simulink model "three_phase_WPT"  (R2020b)
settings: Solver=FixedStepDiscrete  StartTime=0.0  StopTime=Tfinal  FixedStep=SampleTime  RelTol=1e-3
InitFcn:
  | param
values from neighbouring files (symbols this model uses):
  C_DCA = 1e-6    (= 1e-06)    [param.m]
  C_DCB = 1e-6    (= 1e-06)    [param.m]
  C_DCC = 1e-6    (= 1e-06)    [param.m]
  Cp = 1.7349e-08    [param.m]
  Cs = 5.9683e-08    [param.m]
  ESRA = 1e-7    (= 1e-07)    [param.m]
  ESRB = 1e-7    (= 1e-07)    [param.m]
  ESRC = 1e-7    (= 1e-07)    [param.m]
  f_motor = 300    [param.m]
  LA_mid_parasitic = 1e-8    (= 1e-08)    [param.m]
  LA_parasitic = 1e-8    (= 1e-08)    [param.m]
  LAB_parasitic = 1e-8    (= 1e-08)    [param.m]
  LB_mid_parasitic = 1e-8    (= 1e-08)    [param.m]
  LB_parasitic = 1e-8    (= 1e-08)    [param.m]
  LBC_parasitic = 1e-8    (= 1e-08)    [param.m]
  LC_mid_parasitic = 1e-8    (= 1e-08)    [param.m]
  LC_parasitic = 1e-8    (= 1e-08)    [param.m]
  Lp = 2.2813e-04    (= 0.00022813)    [param.m]
  Ls = 6.6315e-05    [param.m]
  LSource = 1e-6    (= 1e-06)    [param.m]
  M = 1.8450e-05    (= 1.845e-05)    [param.m]
  ma = 0:0.01:1    [analitik_calculation.m]    (also in analytical_v2.m; param.m = 0.9)
  RA_mid_parasitic = 1e-3    (= 0.001)    [param.m]
  RA_parasitic = 1e-3    (= 0.001)    [param.m]
  RAB_parasitic = 1e-3    (= 0.001)    [param.m]
  RB_mid_parasitic = 1e-3    (= 0.001)    [param.m]
  RBC_parasitic = 1e-3    (= 0.001)    [param.m]
  RC_mid_parasitic = 1e-3    (= 0.001)    [param.m]
  RL = 8.33*1.2337    (= 10.276721)    [param.m]
  RSource = 0.1    [param.m]
  SampleTime = 1e-8    (= 1e-08)    [param.m]
  Tfinal = 0.05    [param.m]
  VDC = 200    [param.m]
undefined symbols (not defined in the file or in its folder): C_DC, ESLA, ESLB
libraries: powerlib x100, eeStairGenerator x2, eeGeneralControl x1
settings Model: Creator=enes_  LastModifiedBy=enes_
settings DataIOCC: ReturnWorkspaceOutputs=off
settings DebuggingCC: ArithmeticOperatorsInVariantConditions=warning
settings SFSimCC: SimUseLocalCustomCode=off  CustomCodeUndefinedFunction=UseInterfaceOnly
settings RTWCC: RTWUseLocalCustomCode=off

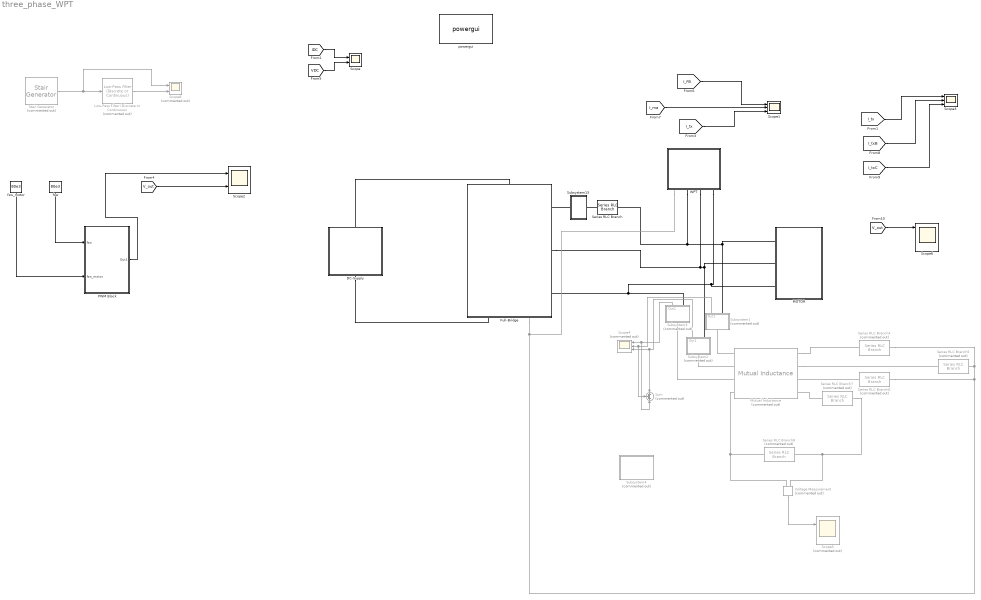
== system three_phase_WPT ==
  DC-Supply : Subsystem
  Full-Bridge : Subsystem
      settings: PortSchema="{\"entries\":[{\"content\":{\"sides\":[{\"content\":{\"connectorIds\":[]},\"type\":\"ConnectorPlacement.EquallySpacedRectSide\",\"uuid\":\"92c2640b-bb56-47f8-9c41-2323b38839f8\"},{\"content\":{\"connectorIds\":[\"RConn1\",\"RConn2\",\"RConn3\"],\"side\":\"RIGHT\"},\"type\":\"ConnectorPlacement.EquallySpacedRectSide\",\"uuid\":\"0b5c90a1-e2e1-4478-84c9-834496a6568e\"},{\"content\":{\"connectorIds\":[\"LConn1\"],\"side\":\"TOP\"},\"type\":\"ConnectorPlacement.EquallySpacedRectSide\",\"uuid\":\"1c803fb0-9096-4a7d-b495-aabd35d72306\"},{\"content\":{\"connectorIds\":[\"RConn4\",\"RConn5\"],\"side\":\"BOTTOM\"},\"type\":\"ConnectorPlacement.EquallySpacedRectSide\",\"uuid\":\"5a2d766c-8c3f-4943-ab0f-0e1988e2f8d8\"},{\"content\":{\"connectorIds\":[],\"side\":\"HIDDEN\"},\"type\":\"ConnectorPlacement.EquallySpacedRectSide\",\"uuid\":\"8868c32c-a67f-4887-a91d-dc24242eaee2\"}]},\"type\":\"ConnectorPlacement.EquallySpacedConnector\",\"uuid\":\"a3546067-6216-40b0-bae0-9d71271c5112\"}],\"packageUris\":[\"http://schema.mathworks.com/mf0/Connector/R2020b\"],\"version\":\"1.0\"}"
  Low-Pass Filter (Discrete or Continuous) : eeGeneralControl/Low-Pass Filter (Discrete or Continuous)  Commented=on  K=1  T=2e-3  B=inf  A=-inf  init_option=Inherited from block input  x0=0  Ts=-1
  MOTOR : Subsystem
      settings: PortSchema="{\"entries\":[{\"content\":{\"sides\":[{\"content\":{\"connectorIds\":[]},\"type\":\"ConnectorPlacement.EquallySpacedRectSide\",\"uuid\":\"27af0988-5d70-46f2-9f63-66e4679735d7\"},{\"content\":{\"connectorIds\":[],\"side\":\"RIGHT\"},\"type\":\"ConnectorPlacement.EquallySpacedRectSide\",\"uuid\":\"9d673fb6-38db-4110-ad66-771dcf318fba\"},{\"content\":{\"connectorIds\":[\"LConn1\",\"LConn2\",\"LConn3\"],\"side\":\"TOP\"},\"type\":\"ConnectorPlacement.EquallySpacedRectSide\",\"uuid\":\"44eb7bd4-c702-4f50-84c2-cb9d75020b5b\"},{\"content\":{\"connectorIds\":[],\"side\":\"HIDDEN\"},\"type\":\"ConnectorPlacement.EquallySpacedRectSide\",\"uuid\":\"ba714e9b-5efc-4dbb-add8-803f06cf9de0\"}]},\"type\":\"ConnectorPlacement.EquallySpacedConnector\",\"uuid\":\"a2219d53-abb4-437b-a840-c37860cec52f\"}],\"packageUris\":[\"http://schema.mathworks.com/mf0/Connector/R2020b\"],\"version\":\"1.0\"}"
  Mutual Inductance : powerlib/Elements/Mutual Inductance  Commented=on  LConnTagsString=a|b|c|L4  RConnTagsString=A|B|C|R4  TypeOfMutual=Generalized mutual inductance  NumberOfWindings=4  SelfImpedance1=[1.1 1.1e-03]  SelfImpedance2=[ 1.1 1.1e-03]  ThreeWindings=on  SelfImpedance3=[ 1.1 1.1e-03]  MutualImpedance=[1.0 1.0e-03]  InductanceMatrix="[1 0  0 0.2 ;  0 1  0 0.2 ;0 0  1 0.2 ;0.2 0.2  0.2 1  ] * 1e-3"  ResistanceMatrix="[ 1  0 0 0 ;  0 1 0 0 ; 0 0 1 0  ;0 0 0 1 ]"  Measurements=Winding currents
      settings: AttributesFormatString=\n  SourceProductBaseCode=PS
  PWM Block : Subsystem
  Scope : Scope  NumInputPorts=2
  Scope1 : Scope  NumInputPorts=3
  Scope2 : Scope  NumInputPorts=2
  Scope3 : Scope  NumInputPorts=3
  Scope4 : Scope  Commented=on  NumInputPorts=3
  Scope5 : Scope  Commented=on  NumInputPorts=2
  Scope6 : Scope  NumInputPorts=3
  Scope8 : Scope  Commented=on  NumInputPorts=2
  Series RLC Branch : powerlib/Elements/Series RLC Branch  LConnTagsString=__new0  RConnTagsString=__new0  BranchType=RL  Resistance=1e-2  Inductance=1e-6  SetiL0=off  InitialCurrent=0  Capacitance=1e-6  Setx0=off  InitialVoltage=0  Measurements=None
  Series RLC Branch4 : powerlib/Elements/Series RLC Branch  Commented=on  LConnTagsString=__new0  RConnTagsString=__new0  BranchType=C  Resistance=1  Inductance=1e-3  SetiL0=off  InitialCurrent=0  Capacitance=3.9579e-09  Setx0=off  InitialVoltage=0  Measurements=None
  Series RLC Branch5 : powerlib/Elements/Series RLC Branch  Commented=on  LConnTagsString=__new0  RConnTagsString=__new0  BranchType=C  Resistance=1  Inductance=1e-3  SetiL0=off  InitialCurrent=0  Capacitance=3.9579e-09  Setx0=off  InitialVoltage=0  Measurements=None
  Series RLC Branch6 : powerlib/Elements/Series RLC Branch  Commented=on  LConnTagsString=__new0  RConnTagsString=__new0  BranchType=C  Resistance=1  Inductance=1e-3  SetiL0=off  InitialCurrent=0  Capacitance=3.9579e-09  Setx0=off  InitialVoltage=0  Measurements=None
  Series RLC Branch7 : powerlib/Elements/Series RLC Branch  Commented=on  LConnTagsString=__new0  RConnTagsString=__new0  BranchType=C  Resistance=1  Inductance=1e-3  SetiL0=off  InitialCurrent=0  Capacitance=Cs  Setx0=off  InitialVoltage=0  Measurements=None
  Series RLC Branch8 : powerlib/Elements/Series RLC Branch  Commented=on  LConnTagsString=__new0  RConnTagsString=__new0  BranchType=R  Resistance=10  Inductance=1e-3  SetiL0=off  InitialCurrent=0  Capacitance=Cs  Setx0=off  InitialVoltage=0  Measurements=None
  Stair Generator : eeStairGenerator/Stair Generator  Commented=on  LabelModeActiveChoice=Discrete  TimeInput=Tfinal*[0 1/4 2/4 3/4 ]  AmplitudeInput=[0.50 0.8 0.6 0.5 ]  SampleTime=-1  RepeatPattern=off  OutDataTypeStr=double
      settings: SourceProductBaseCode=PS
  Subsystem1 : Subsystem  Commented=on
  Subsystem13 : Subsystem
  Subsystem2 : Subsystem  Commented=on
  Subsystem3 : Subsystem  Commented=on
  Subsystem4 : Subsystem  Commented=on
  Sum : Sum  Commented=on  Inputs=+++
  Voltage Measurement : powerlib/Measurements/Voltage Measurement  Commented=on  PhasorSimulation=off  OutputType=Complex  PSBequivalent=0
  WPT : Subsystem
  fsw : Constant  Value=80e3
  fsw_motor : Constant  Value=80e3
  powergui : powerlib/powergui  Priority=1  SimulationMode=Discrete  SampleTime=SampleTime  frequency=60  Iterations=50  frequencyindice=0  Pbase=100e6  ErrMax=1e-4  UnitsV=kV  UnitsW=MW  buscounter=0  FunctionMessages=off  echomessages=off  EnableUseOfTLC=off  CurrentSourceSwitches=off  DisableSnubberDevices=off  DisableRonSwitches=off  DisableVfSwitches=off  DisplayEquations=off  AutomaticDiscreteSolvers=off  SolverType=Tustin/Backward Euler (TBE)  Interpol=off  ExternalGateDelay=off  methode=off  Ts=100  x0status=blocks  SPID=on  SwTol=0  HookPort=off  NonlinearTolerance=1e-4  nMaxIteration=100  ContinueOnMaxIteration=off  RestoreLinks=warning  ResistiveCurrentMeasurement=off  Frange=[1e3:1e3:240e3]  Ylog=off  Xlog=on  ShowGrid=off  save=off  variable=ZData  structure=ScopeData2  ZoomFFT=off  StartTime=0.02  cycles=400  DisplayStyle=2  fundamental=80e3  FreqAxis=off  MaxFrequency=240e3  frequencyindicesteady=1  RmsSteady=1  display=off
  wires:
  Low-Pass Filter (Discrete or Continuous)/1 -> Scope8/2
  [IDC] -> Scope/1
  [VDC] -> Scope/2
  [I_FB] -> Scope1/1
  [I_ma] -> Scope1/2
  [I_tx] -> Scope1/3
  Stair Generator/1 -> Scope8/1, Low-Pass Filter (Discrete or Continuous)/1
  fsw_motor/1 -> PWM Block/2(fsw_motor)
  [V_out] -> Scope2/2
  PWM Block/1(Out1) -> Scope2/1
  fsw/1 -> PWM Block/1(fsw)
  [I_tx] -> Scope3/1
  [I_txB] -> Scope3/2
  [I_txC] -> Scope3/3
  Subsystem3/1(Out1) -> Sum/3, Scope4/1
  Subsystem1/1(Out1) -> Sum/2, Scope4/2
  Subsystem2/1(Out1) -> Sum/1, Scope4/3
  Voltage Measurement/1 -> Scope5/1
  [V_out] -> Scope6/1
  connections:
  DC-Supply/LConn1 -- Full-Bridge/LConn1
  DC-Supply/RConn1 -- Full-Bridge/RConn4
  Series RLC Branch/LConn1 -- Subsystem13/LConn1
  Subsystem13/RConn1 -- Full-Bridge/RConn1
  Full-Bridge/RConn2 -- WPT/LConn2 -- Subsystem2/RConn1 -- MOTOR/LConn2
  Mutual Inductance/RConn2 -- Series RLC Branch5/RConn1
  Series RLC Branch6/RConn1 -- Mutual Inductance/RConn3
  Series RLC Branch7/RConn1 -- Mutual Inductance/RConn4
  Voltage Measurement/LConn1 -- Series RLC Branch7/LConn1 -- Series RLC Branch8/LConn1
  MOTOR/LConn1 -- Series RLC Branch/RConn1 -- WPT/LConn3 -- Subsystem1/RConn1
  Subsystem2/LConn1 -- Mutual Inductance/LConn2
  MOTOR/LConn3 -- WPT/LConn1 -- Full-Bridge/RConn3 -- Subsystem3/RConn1
  Subsystem3/LConn1 -- Mutual Inductance/LConn3
  Mutual Inductance/LConn1 -- Subsystem1/LConn1
  Mutual Inductance/RConn1 -- Series RLC Branch4/RConn1
  Series RLC Branch6/LConn1 -- WPT/LConn4 -- Full-Bridge/RConn5 -- Series RLC Branch4/LConn1 -- Series RLC Branch5/LConn1
  Voltage Measurement/LConn2 -- Mutual Inductance/LConn4 -- Series RLC Branch8/RConn1

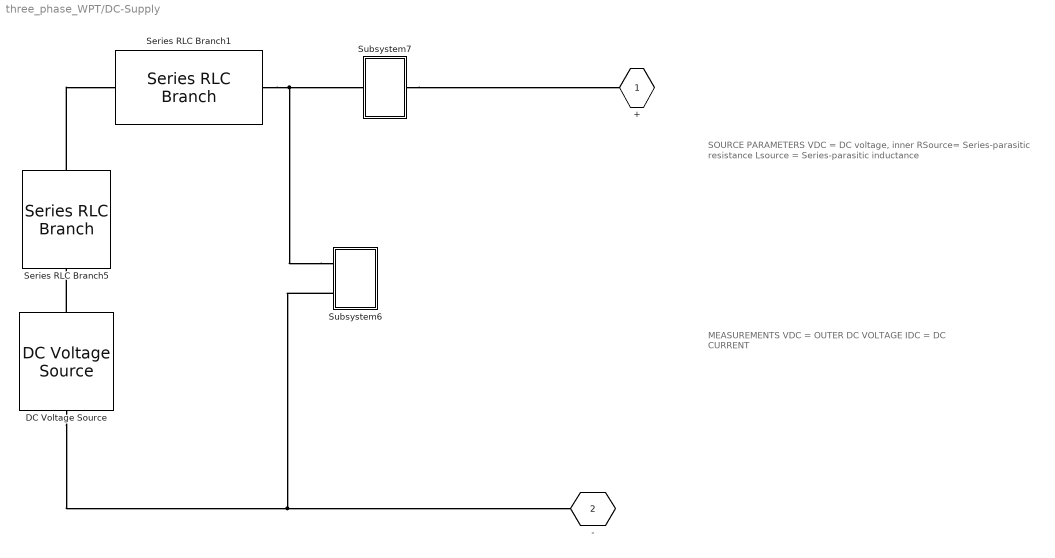
== system three_phase_WPT/DC-Supply ==
  note: SOURCE PARAMETERS
      | VDC = DC voltage, inner
      | RSource= Series-parasitic resistance
      | Lsource = Series-parasitic inductance
  note: MEASUREMENTS
      | VDC = OUTER DC VOLTAGE
      | IDC = DC CURRENT
  DC Voltage Source : powerlib/Electrical Sources/DC Voltage Source  Amplitude=VDC  Measurements=None
  Series RLC Branch1 : powerlib/Elements/Series RLC Branch  LConnTagsString=__new0  RConnTagsString=__new0  BranchType=L  Resistance=LSource  Inductance=LSource  SetiL0=off  InitialCurrent=0  Capacitance=0.01  Setx0=off  InitialVoltage=0  Measurements=None
  Series RLC Branch5 : powerlib/Elements/Series RLC Branch  LConnTagsString=__new0  RConnTagsString=__new0  BranchType=R  Resistance=RSource  Inductance=ESLA  SetiL0=off  InitialCurrent=0  Capacitance=0.01  Setx0=off  InitialVoltage=0  Measurements=None
  Subsystem6 : Subsystem
  Subsystem7 : Subsystem
  + : PMIOPort  Side=Left
  - : PMIOPort  Port=2  Side=Right
  connections:
  Series RLC Branch5/LConn1 -- Series RLC Branch1/RConn1
  DC Voltage Source/LConn1 -- Subsystem6/LConn2 -- -/RConn1
  Subsystem6/LConn1 -- Subsystem7/RConn1 -- Series RLC Branch1/LConn1
  DC Voltage Source/RConn1 -- Series RLC Branch5/RConn1
  Subsystem7/LConn1 -- +/RConn1

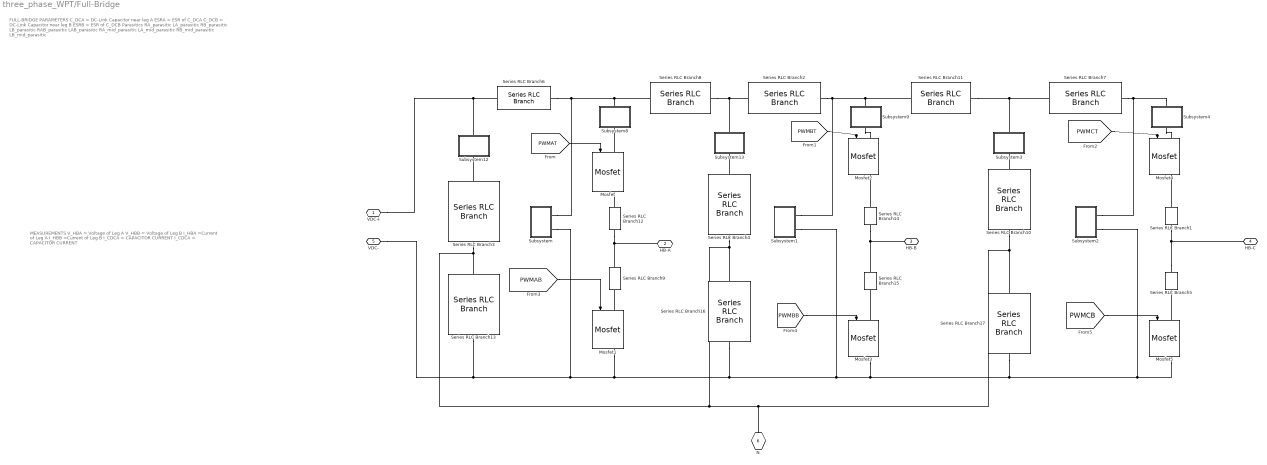
== system three_phase_WPT/Full-Bridge ==
  note: MEASUREMENTS
      | V_HBA = Voltage of Leg A
      | V_HBB = Voltage of Leg B
      | I_HBA =Current of Leg A
      | I_HBB =Current of Leg B
      | I_CDCA = CAPACITOR CURRENT
      | I_CDCA = CAPACITOR CURRENT
  note: FULL-BRIDGE PARAMETERS
      | C_DCA = DC-Link Capacitor near leg A
      | ESRA = ESR of C_DCA
      | C_DCB = DC-Link Capacitor near leg B
      | ESRB = ESR of C_DCB
      | Parasitics
      | RA_parasitic
      | LA_parasitic
      | RB_parasitic
      | LB_parasitic
      | RAB_parasitic
      | LAB_parasitic
      | RA_mid_parasitic
      | LA_mid_parasitic
      | RB_mid_parasitic
      | LB_mid_parasitic
  Mosfet{,1..5} (6 alike) : powerlib/Power Electronics/Mosfet  Ron=0.1  Lon=0  Rd=0.01  Vfd=0  IC=0  Rs=1e5  Cs=inf  Measurements=on
  Series RLC Branch1 : powerlib/Elements/Series RLC Branch  LConnTagsString=__new0  RConnTagsString=__new0  BranchType=RL  Resistance=RC_mid_parasitic  Inductance=LC_mid_parasitic  SetiL0=off  InitialCurrent=0  Capacitance=C_DC  Setx0=off  InitialVoltage=0  Measurements=None
  Series RLC Branch10 : powerlib/Elements/Series RLC Branch  LConnTagsString=__new0  RConnTagsString=__new0  BranchType=RC  Resistance=ESRC  Inductance=ESLB  SetiL0=off  InitialCurrent=0  Capacitance=C_DCC  Setx0=off  InitialVoltage=0  Measurements=None
  Series RLC Branch11 : powerlib/Elements/Series RLC Branch  LConnTagsString=__new0  RConnTagsString=__new0  BranchType=RL  Resistance=RBC_parasitic  Inductance=LBC_parasitic  SetiL0=off  InitialCurrent=0  Capacitance=0.01  Setx0=off  InitialVoltage=0  Measurements=None
  Series RLC Branch12 : powerlib/Elements/Series RLC Branch  LConnTagsString=__new0  RConnTagsString=__new0  BranchType=RL  Resistance=RA_mid_parasitic  Inductance=LA_mid_parasitic  SetiL0=off  InitialCurrent=0  Capacitance=C_DC  Setx0=off  InitialVoltage=0  Measurements=None
  Series RLC Branch13 : powerlib/Elements/Series RLC Branch  LConnTagsString=__new0  RConnTagsString=__new0  BranchType=RC  Resistance=ESRA  Inductance=ESLA  SetiL0=off  InitialCurrent=0  Capacitance=C_DCA  Setx0=off  InitialVoltage=0  Measurements=None
  Series RLC Branch14 : powerlib/Elements/Series RLC Branch  LConnTagsString=__new0  RConnTagsString=__new0  BranchType=RL  Resistance=RB_mid_parasitic  Inductance=LB_mid_parasitic  SetiL0=off  InitialCurrent=0  Capacitance=C_DC  Setx0=off  InitialVoltage=0  Measurements=None
  Series RLC Branch15 : powerlib/Elements/Series RLC Branch  LConnTagsString=__new0  RConnTagsString=__new0  BranchType=RL  Resistance=RB_mid_parasitic  Inductance=LB_mid_parasitic  SetiL0=off  InitialCurrent=0  Capacitance=C_DC  Setx0=off  InitialVoltage=0  Measurements=None
  Series RLC Branch16 : powerlib/Elements/Series RLC Branch  LConnTagsString=__new0  RConnTagsString=__new0  BranchType=RC  Resistance=ESRB  Inductance=ESLB  SetiL0=off  InitialCurrent=0  Capacitance=C_DCB  Setx0=off  InitialVoltage=0  Measurements=None
  Series RLC Branch17 : powerlib/Elements/Series RLC Branch  LConnTagsString=__new0  RConnTagsString=__new0  BranchType=RC  Resistance=ESRB  Inductance=ESLB  SetiL0=off  InitialCurrent=0  Capacitance=C_DCB  Setx0=off  InitialVoltage=0  Measurements=None
  Series RLC Branch2 : powerlib/Elements/Series RLC Branch  LConnTagsString=__new0  RConnTagsString=__new0  BranchType=RL  Resistance=LB_parasitic  Inductance=LB_parasitic  SetiL0=off  InitialCurrent=0  Capacitance=0.01  Setx0=off  InitialVoltage=0  Measurements=None
  Series RLC Branch3 : powerlib/Elements/Series RLC Branch  LConnTagsString=__new0  RConnTagsString=__new0  BranchType=RC  Resistance=ESRA  Inductance=ESLA  SetiL0=off  InitialCurrent=0  Capacitance=C_DCA  Setx0=off  InitialVoltage=0  Measurements=None
  Series RLC Branch4 : powerlib/Elements/Series RLC Branch  LConnTagsString=__new0  RConnTagsString=__new0  BranchType=RC  Resistance=ESRB  Inductance=ESLB  SetiL0=off  InitialCurrent=0  Capacitance=C_DCB  Setx0=off  InitialVoltage=0  Measurements=None
  Series RLC Branch5 : powerlib/Elements/Series RLC Branch  LConnTagsString=__new0  RConnTagsString=__new0  BranchType=RL  Resistance=RC_mid_parasitic  Inductance=LC_mid_parasitic  SetiL0=off  InitialCurrent=0  Capacitance=C_DC  Setx0=off  InitialVoltage=0  Measurements=None
  Series RLC Branch6 : powerlib/Elements/Series RLC Branch  LConnTagsString=__new0  RConnTagsString=__new0  BranchType=RL  Resistance=RA_parasitic  Inductance=LA_parasitic  SetiL0=off  InitialCurrent=0  Capacitance=0.01  Setx0=off  InitialVoltage=0  Measurements=None
  Series RLC Branch7 : powerlib/Elements/Series RLC Branch  LConnTagsString=__new0  RConnTagsString=__new0  BranchType=RL  Resistance=LC_parasitic  Inductance=LC_parasitic  SetiL0=off  InitialCurrent=0  Capacitance=0.01  Setx0=off  InitialVoltage=0  Measurements=None
  Series RLC Branch8 : powerlib/Elements/Series RLC Branch  LConnTagsString=__new0  RConnTagsString=__new0  BranchType=RL  Resistance=RAB_parasitic  Inductance=LAB_parasitic  SetiL0=off  InitialCurrent=0  Capacitance=0.01  Setx0=off  InitialVoltage=0  Measurements=None
  Series RLC Branch9 : powerlib/Elements/Series RLC Branch  LConnTagsString=__new0  RConnTagsString=__new0  BranchType=RL  Resistance=RA_mid_parasitic  Inductance=LA_mid_parasitic  SetiL0=off  InitialCurrent=0  Capacitance=C_DC  Setx0=off  InitialVoltage=0  Measurements=None
  Subsystem : Subsystem
  Subsystem1 : Subsystem
  Subsystem12 : Subsystem
  Subsystem13 : Subsystem
  Subsystem2 : Subsystem
  Subsystem3 : Subsystem
  Subsystem4 : Subsystem
  Subsystem8 : Subsystem
  Subsystem9 : Subsystem
  VDC+ : PMIOPort  Side=Left
  HB-A : PMIOPort  Port=2  Side=Right
  HB-B : PMIOPort  Port=3  Side=Right
  HB-C : PMIOPort  Port=4  Side=Right
  VDC- : PMIOPort  Port=5  Side=Right
  N : PMIOPort  Port=6  Side=Right
  wires:
  [PWMAB] -> Mosfet1/1
  [PWMAT] -> Mosfet/1
  [PWMBB] -> Mosfet3/1
  [PWMBT] -> Mosfet2/1
  [PWMCT] -> Mosfet4/1
  [PWMCB] -> Mosfet5/1
  connections:
  Subsystem13/RConn1 -- Series RLC Branch8/LConn1 -- Series RLC Branch2/RConn1
  VDC+/RConn1 -- Subsystem12/RConn1 -- Series RLC Branch6/RConn1
  Mosfet1/LConn1 -- Series RLC Branch9/LConn1
  Series RLC Branch6/LConn1 -- Subsystem/LConn1 -- Subsystem8/RConn1 -- Series RLC Branch8/RConn1
  Mosfet3/LConn1 -- Series RLC Branch15/LConn1
  Subsystem9/LConn1 -- Mosfet2/LConn1
  Series RLC Branch4/LConn1 -- Subsystem13/LConn1
  Series RLC Branch3/LConn1 -- Subsystem12/LConn1
  Series RLC Branch14/RConn1 -- Mosfet2/RConn1
  Series RLC Branch2/LConn1 -- Subsystem1/LConn1 -- Series RLC Branch11/RConn1 -- Subsystem9/RConn1
  Series RLC Branch12/RConn1 -- Mosfet/RConn1
  Mosfet/LConn1 -- Subsystem8/LConn1
  HB-B/RConn1 -- Series RLC Branch14/LConn1 -- Series RLC Branch15/RConn1
  Series RLC Branch12/LConn1 -- HB-A/RConn1 -- Series RLC Branch9/RConn1
  Subsystem4/RConn1 -- Series RLC Branch7/LConn1 -- Subsystem2/LConn1
  Series RLC Branch5/RConn1 -- HB-C/RConn1 -- Series RLC Branch1/LConn1
  Series RLC Branch11/LConn1 -- Series RLC Branch7/RConn1 -- Subsystem3/RConn1
  Series RLC Branch1/RConn1 -- Mosfet4/RConn1
  Series RLC Branch10/LConn1 -- Subsystem3/LConn1
  Mosfet5/LConn1 -- Series RLC Branch5/LConn1
  Subsystem4/LConn1 -- Mosfet4/LConn1
  Series RLC Branch10/RConn1 -- Series RLC Branch16/LConn1 -- Series RLC Branch4/RConn1 -- Series RLC Branch13/LConn1 -- Series RLC Branch3/RConn1 -- N/RConn1 -- Series RLC Branch17/LConn1
  Series RLC Branch13/RConn1 -- Series RLC Branch16/RConn1 -- Series RLC Branch17/RConn1 -- Subsystem2/LConn2 -- Mosfet5/RConn1 -- Mosfet3/RConn1 -- Subsystem1/LConn2 -- Mosfet1/RConn1 -- Subsystem/LConn2 -- VDC-/RConn1

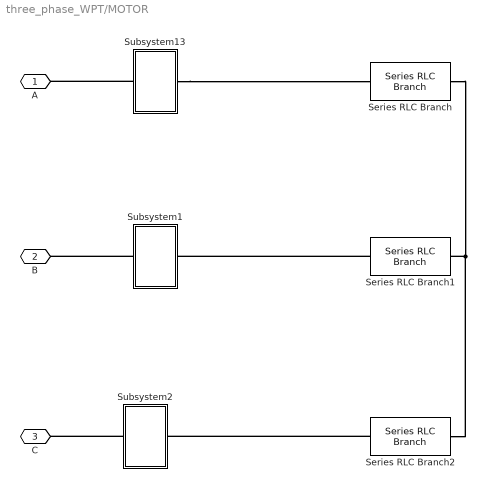
== system three_phase_WPT/MOTOR ==
  Series RLC Branch : powerlib/Elements/Series RLC Branch  LConnTagsString=__new0  RConnTagsString=__new0  BranchType=RL  Resistance=10  Inductance=4e-3  SetiL0=off  InitialCurrent=0  Capacitance=1e-6  Setx0=off  InitialVoltage=0  Measurements=None
  Series RLC Branch1 : powerlib/Elements/Series RLC Branch  LConnTagsString=__new0  RConnTagsString=__new0  BranchType=RL  Resistance=10  Inductance=4e-3  SetiL0=off  InitialCurrent=0  Capacitance=1e-6  Setx0=off  InitialVoltage=0  Measurements=None
  Series RLC Branch2 : powerlib/Elements/Series RLC Branch  LConnTagsString=__new0  RConnTagsString=__new0  BranchType=RL  Resistance=10  Inductance=4e-3  SetiL0=off  InitialCurrent=0  Capacitance=1e-6  Setx0=off  InitialVoltage=0  Measurements=None
  Subsystem1 : Subsystem
  Subsystem13 : Subsystem
  Subsystem2 : Subsystem
  A : PMIOPort  Side=Left
  B : PMIOPort  Port=2  Side=Left
  C : PMIOPort  Port=3  Side=Left
  connections:
  Subsystem13/LConn1 -- Series RLC Branch/LConn1
  Subsystem13/RConn1 -- A/RConn1
  Subsystem1/RConn1 -- B/RConn1
  Subsystem2/RConn1 -- C/RConn1
  Series RLC Branch1/LConn1 -- Subsystem1/LConn1
  Series RLC Branch2/LConn1 -- Subsystem2/LConn1
  Series RLC Branch/RConn1 -- Series RLC Branch2/RConn1 -- Series RLC Branch1/RConn1

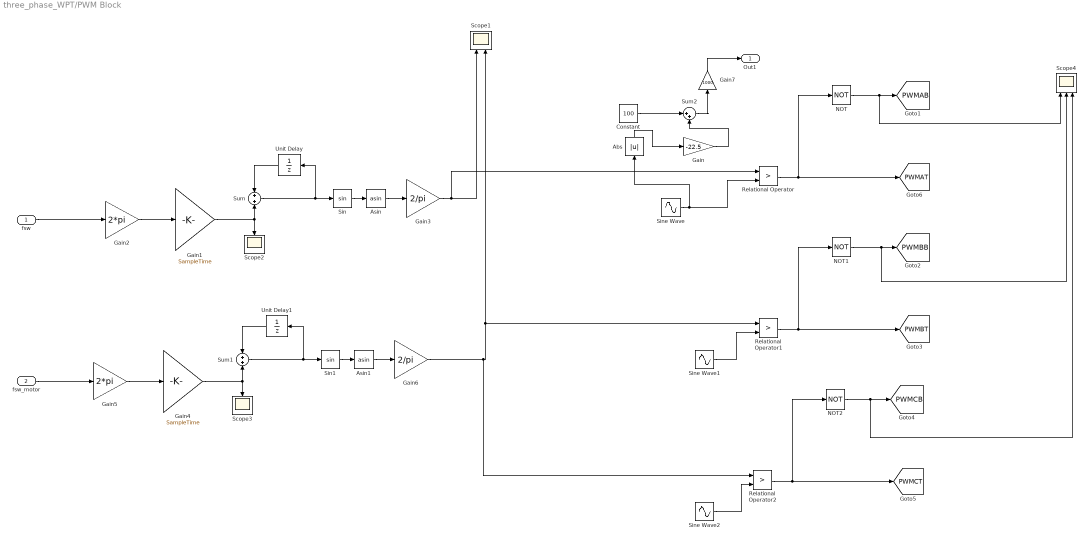
== system three_phase_WPT/PWM Block ==
  fsw : Inport
  fsw_motor : Inport  Port=2
  Abs : Abs
  Asin : Trigonometry  Operator=asin
  Asin1 : Trigonometry  Operator=asin
  Constant : Constant  Value=100
  Gain : Gain  Gain=-22.5
  Gain1 : Gain  Gain=SampleTime
  Gain2 : Gain  Gain=2*pi
  Gain3 : Gain  Gain=2/pi
  Gain4 : Gain  Gain=SampleTime
  Gain5 : Gain  Gain=2*pi
  Gain6 : Gain  Gain=2/pi
  Gain7 : Gain  Gain=1000
  NOT : Logic  Operator=NOT  IconShape=distinctive  AllPortsSameDT=off  OutDataTypeStr=boolean
  NOT1 : Logic  Operator=NOT  IconShape=distinctive  AllPortsSameDT=off  OutDataTypeStr=boolean
  NOT2 : Logic  Operator=NOT  IconShape=distinctive  AllPortsSameDT=off  OutDataTypeStr=boolean
  Relational Operator : RelationalOperator  Operator=>  OutDataTypeStr=boolean  RndMeth=Simplest
  Relational Operator1 : RelationalOperator  Operator=>  OutDataTypeStr=boolean  RndMeth=Simplest
  Relational Operator2 : RelationalOperator  Operator=>  OutDataTypeStr=boolean  RndMeth=Simplest
  Scope1 : Scope  NumInputPorts=2
  Scope2 : Scope
  Scope3 : Scope
  Scope4 : Scope  NumInputPorts=3
  Sin : Trigonometry
  Sin1 : Trigonometry
  Sine Wave : Sin  Amplitude=ma  Frequency=f_motor*2*pi  SampleTime=0
  Sine Wave1 : Sin  Amplitude=ma  Frequency=f_motor*2*pi  Phase=-2*pi/3  SampleTime=0
  Sine Wave2 : Sin  Amplitude=ma  Frequency=f_motor*2*pi  Phase=2*pi/3  SampleTime=0
  Sum : Sum
  Sum1 : Sum
  Sum2 : Sum  Inputs=|++
  Unit Delay : UnitDelay  SampleTime=-1  HasFrameUpgradeWarning=on
  Unit Delay1 : UnitDelay  SampleTime=-1  HasFrameUpgradeWarning=on
  Out1 : Outport
  tag scope: PWMAB=global, PWMAT=global, PWMBB=global, PWMBT=global, PWMCB=global, PWMCT=global
  wires:
  NOT/1 -> Scope4/1, [PWMAB]
  Relational Operator/1 -> NOT/1, [PWMAT]
  Sin/1 -> Asin/1
  Asin/1 -> Gain3/1
  Sum/1 -> Sin/1, Unit Delay/1
  Unit Delay/1 -> Sum/1
  Gain2/1 -> Gain1/1
  Gain1/1 -> Sum/2, Scope2/1
  fsw/1 -> Gain2/1
  Gain6/1 -> Relational Operator2/1, Relational Operator1/1, Scope1/2
  Unit Delay1/1 -> Sum1/1
  Gain4/1 -> Sum1/2, Scope3/1
  Asin1/1 -> Gain6/1
  Sin1/1 -> Asin1/1
  Gain5/1 -> Gain4/1
  fsw_motor/1 -> Gain5/1
  Sum1/1 -> Sin1/1, Unit Delay1/1
  Gain3/1 -> Relational Operator/1, Scope1/1
  Relational Operator1/1 -> NOT1/1, [PWMBT]
  NOT2/1 -> [PWMCB], Scope4/3
  Relational Operator2/1 -> NOT2/1, [PWMCT]
  Sine Wave/1 -> Abs/1, Relational Operator/2
  Sine Wave2/1 -> Relational Operator2/2
  Sine Wave1/1 -> Relational Operator1/2
  NOT1/1 -> Scope4/2, [PWMBB]
  Constant/1 -> Sum2/1
  Gain/1 -> Sum2/2
  Sum2/1 -> Gain7/1
  Gain7/1 -> Out1/1
  Abs/1 -> Gain/1

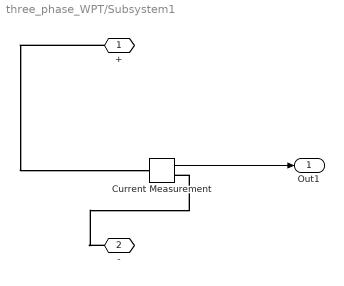
== system three_phase_WPT/Subsystem1 ==
  Current Measurement : powerlib/Measurements/Current Measurement  PhasorSimulation=off  OutputType=Complex  PSBequivalent=0
  + : PMIOPort  Side=Right
  - : PMIOPort  Port=2  Side=Left
  Out1 : Outport
  wires:
  Current Measurement/1 -> Out1/1
  connections:
  +/RConn1 -- Current Measurement/LConn1
  -/RConn1 -- Current Measurement/RConn1

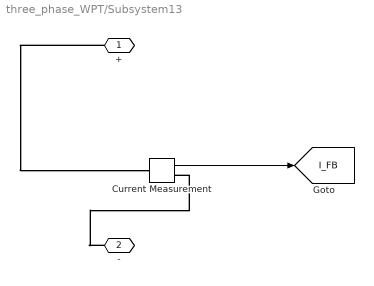
== system three_phase_WPT/Subsystem13 ==
  Current Measurement : powerlib/Measurements/Current Measurement  PhasorSimulation=off  OutputType=Complex  PSBequivalent=0
  + : PMIOPort  Side=Right
  - : PMIOPort  Port=2  Side=Left
  tag scope: I_FB=global
  wires:
  Current Measurement/1 -> [I_FB]
  connections:
  +/RConn1 -- Current Measurement/LConn1
  -/RConn1 -- Current Measurement/RConn1

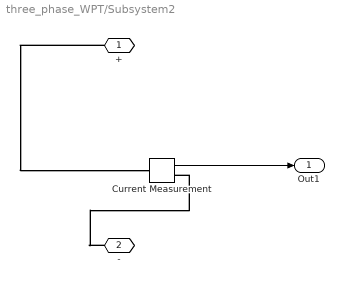
== system three_phase_WPT/Subsystem2 ==
  Current Measurement : powerlib/Measurements/Current Measurement  PhasorSimulation=off  OutputType=Complex  PSBequivalent=0
  + : PMIOPort  Side=Right
  - : PMIOPort  Port=2  Side=Left
  Out1 : Outport
  wires:
  Current Measurement/1 -> Out1/1
  connections:
  +/RConn1 -- Current Measurement/LConn1
  -/RConn1 -- Current Measurement/RConn1

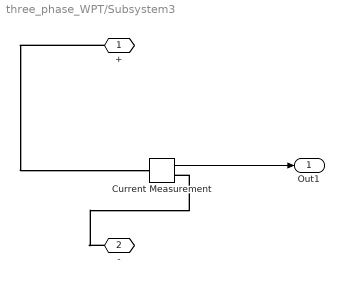
== system three_phase_WPT/Subsystem3 ==
  Current Measurement : powerlib/Measurements/Current Measurement  PhasorSimulation=off  OutputType=Complex  PSBequivalent=0
  + : PMIOPort  Side=Right
  - : PMIOPort  Port=2  Side=Left
  Out1 : Outport
  wires:
  Current Measurement/1 -> Out1/1
  connections:
  +/RConn1 -- Current Measurement/LConn1
  -/RConn1 -- Current Measurement/RConn1

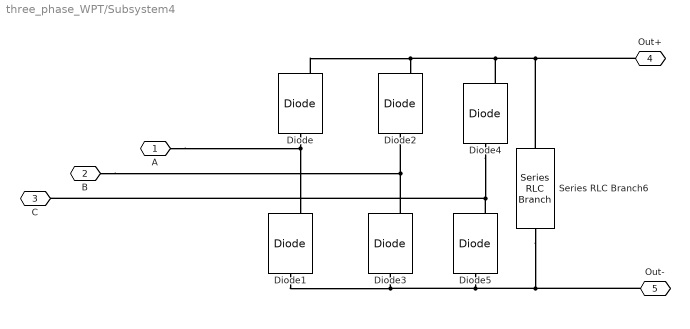
== system three_phase_WPT/Subsystem4 ==
  Diode{,1..5} (6 alike) : powerlib/Power Electronics/Diode  Ron=0.001  Lon=0  Vf=0.8  IC=0  UseSnubber=0  Rs=500  Cs=250e-9  Measurements=on
  Series RLC Branch6 : powerlib/Elements/Series RLC Branch  LConnTagsString=__new0  RConnTagsString=__new0  BranchType=C  Resistance=1  Inductance=1e-3  SetiL0=off  InitialCurrent=0  Capacitance=1e-6  Setx0=off  InitialVoltage=0  Measurements=None
  A : PMIOPort  Side=Left
  B : PMIOPort  Port=2  Side=Left
  C : PMIOPort  Port=3  Side=Left
  Out+ : PMIOPort  Port=4  Side=Right
  Out- : PMIOPort  Port=5  Side=Right
  connections:
  Diode3/RConn1 -- B/RConn1 -- Diode2/LConn1
  Diode/LConn1 -- A/RConn1 -- Diode1/RConn1
  Diode/RConn1 -- Diode2/RConn1 -- Diode4/RConn1 -- Series RLC Branch6/LConn1 -- Out+/RConn1
  Diode1/LConn1 -- Diode3/LConn1 -- Out-/RConn1 -- Series RLC Branch6/RConn1 -- Diode5/LConn1
  Diode4/LConn1 -- C/RConn1 -- Diode5/RConn1

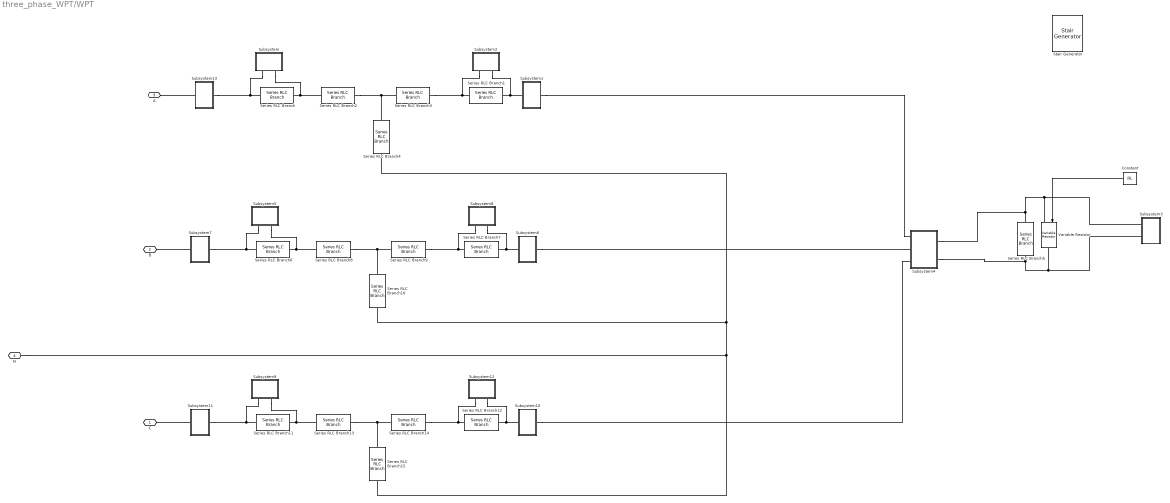
== system three_phase_WPT/WPT ==
  Constant : Constant  Value=RL
  Series RLC Branch : powerlib/Elements/Series RLC Branch  LConnTagsString=__new0  RConnTagsString=__new0  BranchType=C  Resistance=1  Inductance=1e-3  SetiL0=off  InitialCurrent=0  Capacitance=Cp  Setx0=off  InitialVoltage=0  Measurements=None
  Series RLC Branch1 : powerlib/Elements/Series RLC Branch  LConnTagsString=__new0  RConnTagsString=__new0  BranchType=C  Resistance=1  Inductance=1e-3  SetiL0=off  InitialCurrent=0  Capacitance=Cs  Setx0=off  InitialVoltage=0  Measurements=None
  Series RLC Branch{2,4,8,10,13,15} (6 alike) : powerlib/Elements/Series RLC Branch  LConnTagsString=__new0  RConnTagsString=__new0  BranchType=L  Resistance=1  Inductance=Lp-M  SetiL0=off  InitialCurrent=0  Capacitance=Cp  Setx0=off  InitialVoltage=0  Measurements=None
  Series RLC Branch11 : powerlib/Elements/Series RLC Branch  LConnTagsString=__new0  RConnTagsString=__new0  BranchType=C  Resistance=1  Inductance=1e-3  SetiL0=off  InitialCurrent=0  Capacitance=Cp  Setx0=off  InitialVoltage=0  Measurements=None
  Series RLC Branch12 : powerlib/Elements/Series RLC Branch  LConnTagsString=__new0  RConnTagsString=__new0  BranchType=C  Resistance=1  Inductance=1e-3  SetiL0=off  InitialCurrent=0  Capacitance=Cs  Setx0=off  InitialVoltage=0  Measurements=None
  Series RLC Branch14 : powerlib/Elements/Series RLC Branch  LConnTagsString=__new0  RConnTagsString=__new0  BranchType=L  Resistance=1  Inductance=Ls-M  SetiL0=off  InitialCurrent=0  Capacitance=Cp  Setx0=off  InitialVoltage=0  Measurements=None
  Series RLC Branch3 : powerlib/Elements/Series RLC Branch  LConnTagsString=__new0  RConnTagsString=__new0  BranchType=L  Resistance=1  Inductance=Ls-M  SetiL0=off  InitialCurrent=0  Capacitance=Cp  Setx0=off  InitialVoltage=0  Measurements=None
  Series RLC Branch5 : powerlib/Elements/Series RLC Branch  LConnTagsString=__new0  RConnTagsString=__new0  BranchType=R  Resistance=1e6  Inductance=Ls-M  SetiL0=off  InitialCurrent=0  Capacitance=Cp  Setx0=off  InitialVoltage=0  Measurements=None
  Series RLC Branch6 : powerlib/Elements/Series RLC Branch  LConnTagsString=__new0  RConnTagsString=__new0  BranchType=C  Resistance=1  Inductance=1e-3  SetiL0=off  InitialCurrent=0  Capacitance=Cp  Setx0=off  InitialVoltage=0  Measurements=None
  Series RLC Branch7 : powerlib/Elements/Series RLC Branch  LConnTagsString=__new0  RConnTagsString=__new0  BranchType=C  Resistance=1  Inductance=1e-3  SetiL0=off  InitialCurrent=0  Capacitance=Cs  Setx0=off  InitialVoltage=0  Measurements=None
  Series RLC Branch9 : powerlib/Elements/Series RLC Branch  LConnTagsString=__new0  RConnTagsString=__new0  BranchType=L  Resistance=1  Inductance=Ls-M  SetiL0=off  InitialCurrent=0  Capacitance=Cp  Setx0=off  InitialVoltage=0  Measurements=None
  Stair Generator : eeStairGenerator/Stair Generator  LabelModeActiveChoice=Discrete  TimeInput=Tfinal*[0 1/4 2/4 3/4 ]  AmplitudeInput=RL*[1 1/2 0 100 ]  SampleTime=-1  RepeatPattern=off  OutDataTypeStr=double
      settings: SourceProductBaseCode=PS
  Subsystem : Subsystem
  Subsystem1 : Subsystem
  Subsystem10 : Subsystem
  Subsystem11 : Subsystem
  Subsystem12 : Subsystem
  Subsystem13 : Subsystem
  Subsystem2 : Subsystem
  Subsystem3 : Subsystem
  Subsystem4 : Subsystem
  Subsystem5 : Subsystem
  Subsystem6 : Subsystem
  Subsystem7 : Subsystem
  Subsystem8 : Subsystem
  Subsystem9 : Subsystem
  Variable Resistor : powerlib/Elements/Variable Resistor  Rabsmin=1e-3
      settings: SourceProductBaseCode=PS
  C : PMIOPort  Side=Left
  B : PMIOPort  Port=2  Side=Left
  A : PMIOPort  Port=3  Side=Left
  N : PMIOPort  Port=4  Side=Left
  wires:
  Constant/1 -> Variable Resistor/1
  connections:
  Subsystem13/LConn1 -- Subsystem/LConn1 -- Series RLC Branch/LConn1
  Subsystem13/RConn1 -- A/RConn1
  Series RLC Branch2/LConn1 -- Subsystem/LConn2 -- Series RLC Branch/RConn1
  Series RLC Branch3/RConn1 -- Subsystem2/LConn1 -- Series RLC Branch1/RConn1
  Series RLC Branch4/LConn1 -- Series RLC Branch2/RConn1 -- Series RLC Branch3/LConn1
  Subsystem3/LConn1 -- Variable Resistor/LConn1 -- Series RLC Branch5/LConn1 -- Subsystem4/RConn1
  Subsystem1/RConn1 -- Subsystem2/LConn2 -- Series RLC Branch1/LConn1
  Subsystem3/LConn2 -- Subsystem4/RConn2 -- Series RLC Branch5/RConn1 -- Variable Resistor/RConn1
  Subsystem8/LConn1 -- Series RLC Branch7/RConn1 -- Series RLC Branch9/RConn1
  Subsystem5/LConn1 -- Series RLC Branch6/LConn1 -- Subsystem7/LConn1
  Subsystem5/LConn2 -- Series RLC Branch6/RConn1 -- Series RLC Branch8/LConn1
  Series RLC Branch8/RConn1 -- Series RLC Branch9/LConn1 -- Series RLC Branch10/LConn1
  Subsystem8/LConn2 -- Series RLC Branch7/LConn1 -- Subsystem6/RConn1
  Subsystem6/LConn1 -- Subsystem4/LConn2
  Subsystem7/RConn1 -- B/RConn1
  Subsystem12/LConn1 -- Series RLC Branch12/RConn1 -- Series RLC Branch14/RConn1
  Series RLC Branch4/RConn1 -- Series RLC Branch10/RConn1 -- N/RConn1 -- Series RLC Branch15/RConn1
  Subsystem9/LConn1 -- Series RLC Branch11/LConn1 -- Subsystem11/LConn1
  Subsystem9/LConn2 -- Series RLC Branch11/RConn1 -- Series RLC Branch13/LConn1
  Series RLC Branch13/RConn1 -- Series RLC Branch14/LConn1 -- Series RLC Branch15/LConn1
  Subsystem12/LConn2 -- Series RLC Branch12/LConn1 -- Subsystem10/RConn1
  Subsystem10/LConn1 -- Subsystem4/LConn3
  Subsystem11/RConn1 -- C/RConn1
  Subsystem1/LConn1 -- Subsystem4/LConn1

== system three_phase_WPT/DC-Supply/Subsystem6 ==
  Voltage Measurement : powerlib/Measurements/Voltage Measurement  PhasorSimulation=off  OutputType=Complex  PSBequivalent=0
  + : PMIOPort  Side=Left
  - : PMIOPort  Port=2  Side=Left
  tag scope: VDC=global
  wires:
  Voltage Measurement/1 -> [VDC]
  connections:
  Voltage Measurement/LConn1 -- +/RConn1
  Voltage Measurement/LConn2 -- -/RConn1

== system three_phase_WPT/DC-Supply/Subsystem7 ==
  Current Measurement : powerlib/Measurements/Current Measurement  PhasorSimulation=off  OutputType=Complex  PSBequivalent=0
  + : PMIOPort  Side=Right
  - : PMIOPort  Port=2  Side=Left
  tag scope: IDC=global
  wires:
  Current Measurement/1 -> [IDC]
  connections:
  +/RConn1 -- Current Measurement/LConn1
  -/RConn1 -- Current Measurement/RConn1

== system three_phase_WPT/Full-Bridge/Subsystem ==
  Voltage Measurement : powerlib/Measurements/Voltage Measurement  PhasorSimulation=off  OutputType=Complex  PSBequivalent=0
  + : PMIOPort  Side=Left
  - : PMIOPort  Port=2  Side=Left
  tag scope: V_HBA=global
  wires:
  Voltage Measurement/1 -> [V_HBA]
  connections:
  Voltage Measurement/LConn1 -- +/RConn1
  Voltage Measurement/LConn2 -- -/RConn1

== system three_phase_WPT/Full-Bridge/Subsystem1 ==
  Voltage Measurement : powerlib/Measurements/Voltage Measurement  PhasorSimulation=off  OutputType=Complex  PSBequivalent=0
  + : PMIOPort  Side=Left
  - : PMIOPort  Port=2  Side=Left
  tag scope: V_HBB=global
  wires:
  Voltage Measurement/1 -> [V_HBB]
  connections:
  Voltage Measurement/LConn1 -- +/RConn1
  Voltage Measurement/LConn2 -- -/RConn1

== system three_phase_WPT/Full-Bridge/Subsystem12 ==
  Current Measurement : powerlib/Measurements/Current Measurement  PhasorSimulation=off  OutputType=Complex  PSBequivalent=0
  + : PMIOPort  Side=Right
  - : PMIOPort  Port=2  Side=Left
  tag scope: IC_DCA=global
  wires:
  Current Measurement/1 -> [IC_DCA]
  connections:
  +/RConn1 -- Current Measurement/LConn1
  -/RConn1 -- Current Measurement/RConn1

== system three_phase_WPT/Full-Bridge/Subsystem13 ==
  Current Measurement : powerlib/Measurements/Current Measurement  PhasorSimulation=off  OutputType=Complex  PSBequivalent=0
  + : PMIOPort  Side=Right
  - : PMIOPort  Port=2  Side=Left
  tag scope: I_CDCB=global
  wires:
  Current Measurement/1 -> [I_CDCB]
  connections:
  +/RConn1 -- Current Measurement/LConn1
  -/RConn1 -- Current Measurement/RConn1

== system three_phase_WPT/Full-Bridge/Subsystem2 ==
  Voltage Measurement : powerlib/Measurements/Voltage Measurement  PhasorSimulation=off  OutputType=Complex  PSBequivalent=0
  + : PMIOPort  Side=Left
  - : PMIOPort  Port=2  Side=Left
  tag scope: V_HBC=global
  wires:
  Voltage Measurement/1 -> [V_HBC]
  connections:
  Voltage Measurement/LConn1 -- +/RConn1
  Voltage Measurement/LConn2 -- -/RConn1

== system three_phase_WPT/Full-Bridge/Subsystem3 ==
  Current Measurement : powerlib/Measurements/Current Measurement  PhasorSimulation=off  OutputType=Complex  PSBequivalent=0
  + : PMIOPort  Side=Right
  - : PMIOPort  Port=2  Side=Left
  tag scope: I_CDCC=global
  wires:
  Current Measurement/1 -> [I_CDCC]
  connections:
  +/RConn1 -- Current Measurement/LConn1
  -/RConn1 -- Current Measurement/RConn1

== system three_phase_WPT/Full-Bridge/Subsystem4 ==
  Current Measurement : powerlib/Measurements/Current Measurement  PhasorSimulation=off  OutputType=Complex  PSBequivalent=0
  + : PMIOPort  Side=Right
  - : PMIOPort  Port=2  Side=Left
  tag scope: I_HBC=global
  wires:
  Current Measurement/1 -> [I_HBC]
  connections:
  +/RConn1 -- Current Measurement/LConn1
  -/RConn1 -- Current Measurement/RConn1

== system three_phase_WPT/Full-Bridge/Subsystem8 ==
  Current Measurement : powerlib/Measurements/Current Measurement  PhasorSimulation=off  OutputType=Complex  PSBequivalent=0
  + : PMIOPort  Side=Right
  - : PMIOPort  Port=2  Side=Left
  tag scope: I_HBA=global
  wires:
  Current Measurement/1 -> [I_HBA]
  connections:
  +/RConn1 -- Current Measurement/LConn1
  -/RConn1 -- Current Measurement/RConn1

== system three_phase_WPT/Full-Bridge/Subsystem9 ==
  Current Measurement : powerlib/Measurements/Current Measurement  PhasorSimulation=off  OutputType=Complex  PSBequivalent=0
  + : PMIOPort  Side=Right
  - : PMIOPort  Port=2  Side=Left
  tag scope: I_HBB=global
  wires:
  Current Measurement/1 -> [I_HBB]
  connections:
  +/RConn1 -- Current Measurement/LConn1
  -/RConn1 -- Current Measurement/RConn1

== system three_phase_WPT/MOTOR/Subsystem1 ==
  Current Measurement : powerlib/Measurements/Current Measurement  PhasorSimulation=off  OutputType=Complex  PSBequivalent=0
  + : PMIOPort  Side=Right
  - : PMIOPort  Port=2  Side=Left
  tag scope: I_mb=global
  wires:
  Current Measurement/1 -> [I_mb]
  connections:
  +/RConn1 -- Current Measurement/LConn1
  -/RConn1 -- Current Measurement/RConn1

== system three_phase_WPT/MOTOR/Subsystem13 ==
  Current Measurement : powerlib/Measurements/Current Measurement  PhasorSimulation=off  OutputType=Complex  PSBequivalent=0
  + : PMIOPort  Side=Right
  - : PMIOPort  Port=2  Side=Left
  tag scope: I_ma=global
  wires:
  Current Measurement/1 -> [I_ma]
  connections:
  +/RConn1 -- Current Measurement/LConn1
  -/RConn1 -- Current Measurement/RConn1

== system three_phase_WPT/MOTOR/Subsystem2 ==
  Current Measurement : powerlib/Measurements/Current Measurement  PhasorSimulation=off  OutputType=Complex  PSBequivalent=0
  + : PMIOPort  Side=Right
  - : PMIOPort  Port=2  Side=Left
  tag scope: I_mc=global
  wires:
  Current Measurement/1 -> [I_mc]
  connections:
  +/RConn1 -- Current Measurement/LConn1
  -/RConn1 -- Current Measurement/RConn1

== system three_phase_WPT/WPT/Subsystem ==
  Voltage Measurement : powerlib/Measurements/Voltage Measurement  PhasorSimulation=off  OutputType=Complex  PSBequivalent=0
  + : PMIOPort  Side=Left
  - : PMIOPort  Port=2  Side=Left
  tag scope: V_txCap=global
  wires:
  Voltage Measurement/1 -> [V_txCap]
  connections:
  Voltage Measurement/LConn1 -- +/RConn1
  Voltage Measurement/LConn2 -- -/RConn1

== system three_phase_WPT/WPT/Subsystem1 ==
  Current Measurement : powerlib/Measurements/Current Measurement  PhasorSimulation=off  OutputType=Complex  PSBequivalent=0
  + : PMIOPort  Side=Right
  - : PMIOPort  Port=2  Side=Left
  tag scope: I_rx=global
  wires:
  Current Measurement/1 -> [I_rx]
  connections:
  +/RConn1 -- Current Measurement/LConn1
  -/RConn1 -- Current Measurement/RConn1

== system three_phase_WPT/WPT/Subsystem10 ==
  Current Measurement : powerlib/Measurements/Current Measurement  PhasorSimulation=off  OutputType=Complex  PSBequivalent=0
  + : PMIOPort  Side=Right
  - : PMIOPort  Port=2  Side=Left
  tag scope: I_rxC=global
  wires:
  Current Measurement/1 -> [I_rxC]
  connections:
  +/RConn1 -- Current Measurement/LConn1
  -/RConn1 -- Current Measurement/RConn1

== system three_phase_WPT/WPT/Subsystem11 ==
  Current Measurement : powerlib/Measurements/Current Measurement  PhasorSimulation=off  OutputType=Complex  PSBequivalent=0
  + : PMIOPort  Side=Right
  - : PMIOPort  Port=2  Side=Left
  tag scope: I_txC=global
  wires:
  Current Measurement/1 -> [I_txC]
  connections:
  +/RConn1 -- Current Measurement/LConn1
  -/RConn1 -- Current Measurement/RConn1

== system three_phase_WPT/WPT/Subsystem12 ==
  Voltage Measurement : powerlib/Measurements/Voltage Measurement  PhasorSimulation=off  OutputType=Complex  PSBequivalent=0
  + : PMIOPort  Side=Left
  - : PMIOPort  Port=2  Side=Left
  tag scope: V_rxCapC=global
  wires:
  Voltage Measurement/1 -> [V_rxCapC]
  connections:
  Voltage Measurement/LConn1 -- +/RConn1
  Voltage Measurement/LConn2 -- -/RConn1

== system three_phase_WPT/WPT/Subsystem13 ==
  Current Measurement : powerlib/Measurements/Current Measurement  PhasorSimulation=off  OutputType=Complex  PSBequivalent=0
  + : PMIOPort  Side=Right
  - : PMIOPort  Port=2  Side=Left
  tag scope: I_tx=global
  wires:
  Current Measurement/1 -> [I_tx]
  connections:
  +/RConn1 -- Current Measurement/LConn1
  -/RConn1 -- Current Measurement/RConn1

== system three_phase_WPT/WPT/Subsystem2 ==
  Voltage Measurement : powerlib/Measurements/Voltage Measurement  PhasorSimulation=off  OutputType=Complex  PSBequivalent=0
  + : PMIOPort  Side=Left
  - : PMIOPort  Port=2  Side=Left
  tag scope: V_rxCap=global
  wires:
  Voltage Measurement/1 -> [V_rxCap]
  connections:
  Voltage Measurement/LConn1 -- +/RConn1
  Voltage Measurement/LConn2 -- -/RConn1

== system three_phase_WPT/WPT/Subsystem3 ==
  Voltage Measurement : powerlib/Measurements/Voltage Measurement  PhasorSimulation=off  OutputType=Complex  PSBequivalent=0
  + : PMIOPort  Side=Left
  - : PMIOPort  Port=2  Side=Left
  tag scope: V_out=global
  wires:
  Voltage Measurement/1 -> [V_out]
  connections:
  Voltage Measurement/LConn1 -- +/RConn1
  Voltage Measurement/LConn2 -- -/RConn1

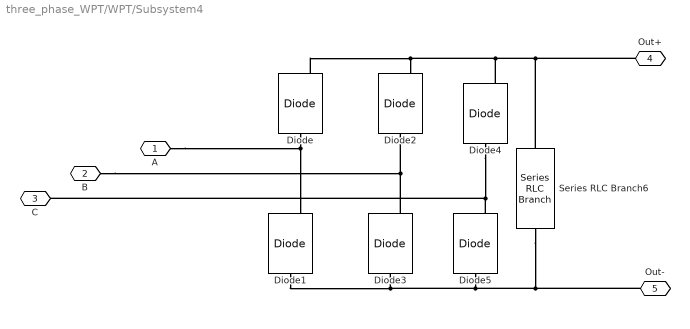
== system three_phase_WPT/WPT/Subsystem4 ==
  Diode{,1..5} (6 alike) : powerlib/Power Electronics/Diode  Ron=0.001  Lon=0  Vf=0.8  IC=0  UseSnubber=0  Rs=500  Cs=250e-9  Measurements=on
  Series RLC Branch6 : powerlib/Elements/Series RLC Branch  LConnTagsString=__new0  RConnTagsString=__new0  BranchType=C  Resistance=1  Inductance=1e-3  SetiL0=off  InitialCurrent=0  Capacitance=1e-6  Setx0=off  InitialVoltage=0  Measurements=None
  A : PMIOPort  Side=Left
  B : PMIOPort  Port=2  Side=Left
  C : PMIOPort  Port=3  Side=Left
  Out+ : PMIOPort  Port=4  Side=Right
  Out- : PMIOPort  Port=5  Side=Right
  connections:
  Diode3/RConn1 -- B/RConn1 -- Diode2/LConn1
  Diode/LConn1 -- A/RConn1 -- Diode1/RConn1
  Diode/RConn1 -- Diode2/RConn1 -- Diode4/RConn1 -- Series RLC Branch6/LConn1 -- Out+/RConn1
  Diode1/LConn1 -- Diode3/LConn1 -- Out-/RConn1 -- Series RLC Branch6/RConn1 -- Diode5/LConn1
  Diode4/LConn1 -- C/RConn1 -- Diode5/RConn1

== system three_phase_WPT/WPT/Subsystem5 ==
  Voltage Measurement : powerlib/Measurements/Voltage Measurement  PhasorSimulation=off  OutputType=Complex  PSBequivalent=0
  + : PMIOPort  Side=Left
  - : PMIOPort  Port=2  Side=Left
  tag scope: V_txCapB=global
  wires:
  Voltage Measurement/1 -> [V_txCapB]
  connections:
  Voltage Measurement/LConn1 -- +/RConn1
  Voltage Measurement/LConn2 -- -/RConn1

== system three_phase_WPT/WPT/Subsystem6 ==
  Current Measurement : powerlib/Measurements/Current Measurement  PhasorSimulation=off  OutputType=Complex  PSBequivalent=0
  + : PMIOPort  Side=Right
  - : PMIOPort  Port=2  Side=Left
  tag scope: I_rxB=global
  wires:
  Current Measurement/1 -> [I_rxB]
  connections:
  +/RConn1 -- Current Measurement/LConn1
  -/RConn1 -- Current Measurement/RConn1

== system three_phase_WPT/WPT/Subsystem7 ==
  Current Measurement : powerlib/Measurements/Current Measurement  PhasorSimulation=off  OutputType=Complex  PSBequivalent=0
  + : PMIOPort  Side=Right
  - : PMIOPort  Port=2  Side=Left
  tag scope: I_txB=global
  wires:
  Current Measurement/1 -> [I_txB]
  connections:
  +/RConn1 -- Current Measurement/LConn1
  -/RConn1 -- Current Measurement/RConn1

== system three_phase_WPT/WPT/Subsystem8 ==
  Voltage Measurement : powerlib/Measurements/Voltage Measurement  PhasorSimulation=off  OutputType=Complex  PSBequivalent=0
  + : PMIOPort  Side=Left
  - : PMIOPort  Port=2  Side=Left
  tag scope: V_rxCapB=global
  wires:
  Voltage Measurement/1 -> [V_rxCapB]
  connections:
  Voltage Measurement/LConn1 -- +/RConn1
  Voltage Measurement/LConn2 -- -/RConn1

== system three_phase_WPT/WPT/Subsystem9 ==
  Voltage Measurement : powerlib/Measurements/Voltage Measurement  PhasorSimulation=off  OutputType=Complex  PSBequivalent=0
  + : PMIOPort  Side=Left
  - : PMIOPort  Port=2  Side=Left
  tag scope: V_txCapC=global
  wires:
  Voltage Measurement/1 -> [V_txCapC]
  connections:
  Voltage Measurement/LConn1 -- +/RConn1
  Voltage Measurement/LConn2 -- -/RConn1
